simulink model "PhaseII_opalrt_NoProtection"  (Simulink 8.8)
settings: Solver=ode3  StartTime=0.0  StopTime=inf  FixedStep=Ts  RelTol=1e-5  EnableMultiTasking=on
PostLoadFcn:
  | %BESS ctrl
  | Kpf=0.005*3*12;
  | Kif=5*6;
  | 
  | Kpf1=0.005*3*12;
  | Kif1=5*6;
  | Kp_v=0.016*15*35;
  | Ki_v=12*25;
  | 
  | Kp_v1=0.016*15*35;
  | Ki_v1=12*25;
  | 
  | Vabc_B=12.47e3;
  | Vdc_ref=Vabc_B*2;
  | Kpwm=sqrt(2)*Vabc_B/Vdc_ref;
  | ZB=Vabc_B^2/1e6;
  | R=0.005*ZB;
  | Ibasefull=673/2*sqrt(2);
  | 
  | 
  | Ts_Control=1e-4;
  | ts=0.05;
  | delay=0.2;
  | offset=10e3;
  | t_plan=60;
  | t_monitor=.2;
  | t_mon=t_monitor;
  | scalingfactor=1;
  | x=0.5;
  | n=6;
  | %t_plan=1/15;
  | %t_monitor=10/900;
  | %t_mon=10/900;
  | 
  | %t_plan=1/5;
  | %t_monitor=10/300;
  | %t_mon=10/300;
  | %scalingfactor=1/300;
  | 
  | f0=60;
  | 
  | Pabc_B=1e6;
  | Iabc_B=Pabc_B*sqrt(2/3)/Vabc_B;  % pk value
  | Imax_1=2.5;
  | Ptrans_B=Pabc_B*200;
  | 
  | Vdc_ref=Vabc_B*2;
  | 
  | ZB=Vabc_B^2/Pabc_B;
  | L=0.1*ZB/2/pi/60;
  | R=0.1*ZB;
  | C=1/(4*pi^2*(2e3)^2*L);
  | 
  | LL=0.005*ZB/2/pi/60;
  | RR=0.005*ZB;
  | 
  | RC=0.02;
  | 
  | %%% Initial SOC %%%%
  | SOC_ini_BESS1=0.5;
  | ... (+223 lines)
InitFcn:
  | %BESS ctrl
  | Kpf=0.005*3*12;
  | Kif=5*6;
  | 
  | Kpf1=0.005*3*12;
  | Kif1=5*6;
  | Kp_v=0.016*15*35;
  | Ki_v=12*25;
  | 
  | Kp_v1=0.016*15*35;
  | Ki_v1=12*25;
  | 
  | Vabc_B=12.47e3;
  | Vdc_ref=Vabc_B*2;
  | Kpwm=sqrt(2)*Vabc_B/Vdc_ref;
  | ZB=Vabc_B^2/1e6;
  | R=0.005*ZB;
  | Ibasefull=673/2*sqrt(2);
  | 
  | 
  | Ts_Control=1e-4;
  | ts=0.05;
  | delay=0.2;
  | offset=10e3;
  | t_plan=60;
  | t_monitor=.2;
  | t_mon=t_monitor;
  | scalingfactor=1;
  | x=0.5;
  | n=6;
  | %t_plan=1/15;
  | %t_monitor=10/900;
  | %t_mon=10/900;
  | 
  | %t_plan=1/5;
  | %t_monitor=10/300;
  | %t_mon=10/300;
  | %scalingfactor=1/300;
  | 
  | f0=60;
  | 
  | Pabc_B=1e6;
  | Iabc_B=Pabc_B*sqrt(2/3)/Vabc_B;  % pk value
  | Imax_1=2.5;
  | Ptrans_B=Pabc_B*200;
  | 
  | Vdc_ref=Vabc_B*2;
  | 
  | ZB=Vabc_B^2/Pabc_B;
  | L=0.1*ZB/2/pi/60;
  | R=0.1*ZB;
  | C=1/(4*pi^2*(2e3)^2*L);
  | 
  | LL=0.005*ZB/2/pi/60;
  | RR=0.005*ZB;
  | 
  | RC=0.02;
  | 
  | %%% Initial SOC %%%%
  | SOC_ini_BESS1=0.5;
  | ... (+223 lines)
undefined symbols (not defined in the file): D1, Delta, DiscIntNeverNeededParam, Left, PG2ref, type, V
libraries: powerlib x220, powerlib_meascontrol x82, dspstat3 x54, dsparch4 x43, dspswit3 x24, simulink x19, simulink_extras x12, powerlib_extras x11, ssn_lib x7, artemis x6, rtlab x5, rtio_generic_dnp3 x5
(part 8 of 9)

== system PhaseII_opalrt_NoProtection/SS_LocalControl/BESS2/Sequence decomposition2 ==
  abc : Inport
  Phase : Inport  Port=2
  Add : Sum  Inputs=+++
  Add1 : Sum
  Add2 : Sum  Inputs=+-
  Add3 : Sum
  Add4 : Sum  Inputs=-+
  Alpha-Beta-Zero to dq0 : powerlib_meascontrol/Transformations/Alpha-Beta-Zero to dq0  Alignment=90 degrees behind phase A axis
  Alpha-Beta-Zero to dq1 : powerlib_meascontrol/Transformations/Alpha-Beta-Zero to dq0  Alignment=90 degrees behind phase A axis
  Delay : Delay  DelayLength=42  InitialCondition=0
  Delay1 : Delay  DelayLength=42  InitialCondition=0
  Demux1 : Demux  Outputs=2
  Demux4 : Demux  Outputs=3
  Fcn3 : Fcn  Expr=sqrt(2/3)*(u[1]-u[2]*1/2-u[3]*1/2)
  Fcn5 : Fcn  Expr=sqrt(2/3)*(u[2]*sqrt(3)/2-u[3]*sqrt(3)/2)
  Gain1 : Gain  Gain=-1
  Gain2 : Gain  Gain=1/3
  Gain3 : Gain
  Gain{6..9} (4 alike) : Gain  Gain=1/2
  Mux : Mux  Inputs=3
  Mux1 : Mux  Inputs=3
  Mux2 : Mux  Inputs=2
  Mux3 : Mux  Inputs=3
  Pos_dq : Outport
  Neg_dq : Outport  Port=2
  zero : Outport  Port=3
  wires:
  Demux1/1 -> Add2/1, Add3/1, Delay/1
  Mux2/1 -> Demux1/1
  Demux1/2 -> Delay1/1, Add4/2, Add1/1
  Mux/1 -> Alpha-Beta-Zero to dq1/1
  Gain1/1 -> Alpha-Beta-Zero to dq1/2
  Alpha-Beta-Zero to dq0/1 -> Pos_dq/1
  Alpha-Beta-Zero to dq1/1 -> Neg_dq/1
  abc/1 -> Demux4/1
  Demux4/1 -> Mux1/1, Add/1
  Demux4/2 -> Mux1/2, Add/3
  Demux4/3 -> Mux1/3, Add/2
  Delay1/1 -> Add2/2, Add3/2
  Delay/1 -> Add4/1, Add1/2
  Add1/1 -> Gain7/1
  Add2/1 -> Gain6/1
  Add4/1 -> Gain9/1
  Add3/1 -> Gain8/1
  Gain8/1 -> Mux/1
  Gain9/1 -> Mux/2
  Mux3/1 -> Alpha-Beta-Zero to dq0/1
  Gain6/1 -> Mux3/1
  Gain7/1 -> Mux3/2
  Add/1 -> Gain2/1, Gain3/1
  Gain2/1 -> zero/1
  Phase/1 -> Gain1/1, Alpha-Beta-Zero to dq0/2
  Gain3/1 -> Mux3/3, Mux/3
  Mux1/1 -> Fcn3/1, Fcn5/1
  Fcn3/1 -> Mux2/1
  Fcn5/1 -> Mux2/2

== system PhaseII_opalrt_NoProtection/SS_LocalControl/BESS2/Subsystem ==
  I_RMS : Inport
  Add : Sum  Inputs=+-
  Constant : Constant  Value=SOC_ini_BESS2*AH*3600
  Constant1 : Constant
  Gain : Gain  Gain=1/3600
  Gain3 : Gain  Gain=1/(AH*3600)
  Gain8 : Gain
  Integrator : Integrator
  Integrator1 : Integrator  InitialConditionSource=external  LimitOutput=on  UpperSaturationLimit=AH*3600  LowerSaturationLimit=0
  Battery_Ah : Outport
  Battery_SOC : Outport  Port=2
  wires:
  Gain8/1 -> Battery_SOC/1
  Gain/1 -> Battery_Ah/1
  I_RMS/1 -> Integrator1/1, Integrator/1
  Constant/1 -> Integrator1/2
  Add/1 -> Gain8/1
  Constant1/1 -> Add/1
  Gain3/1 -> Add/2
  Integrator1/1 -> Gain3/1
  Integrator/1 -> Gain/1

== system PhaseII_opalrt_NoProtection/SS_LocalControl/BESS2/V_theta_generation ==
  Pin : Inport
  Qin : Inport  Port=2
  Pin1 : Inport  Port=3
  "  " : Constant  Value=2*pi
  2 kHz1 : dsparch4/Analog Filter Design  method=Butterworth  filttype=Lowpass  N=2  Wlo=2*pi*0.1  Whi=80  Rp=2  Rs=40
  Constant1 : Constant  Value=1.64368  OutDataTypeStr=single
  D1 : Scope  Commented=on
  D{2..7} (6 alike) : Scope
  Delay : Delay  DelayLength=1  SampleTime=Ts
  Gain1 : Gain
  Gain2 : Gain  Gain=2*pi
  Gain3 : Gain
  Gain4 : Gain  Gain=1/2/pi
  Gain5 : Gain  Gain=1/2/pi
  Gain6 : Gain  Gain=0
  Gain7 : Gain  Gain=1/2/pi
  Gain8 : Gain  Gain=0
  Integrator : Integrator  ExternalReset=rising  InitialConditionSource=external  LimitOutput=on
  Kv : Constant  Value=0.1
  Math Function : Math  Operator=mod  SaturateOnIntegerOverflow=on
  P1 : Constant  Value=0.5
  P4 : Constant  Value=0
  P5 : Constant  Value=0.01
  Product : Product
  Product1 : Product
  Product2 : Product
  Q : Constant  Value=0
  Sum1 : Sum  Inputs=|-+
  Sum10 : Sum  Inputs=|++
  Sum13 : Sum  Inputs=+++
  Sum2 : Sum  Inputs=++++
  Sum3 : Sum  Inputs=|-+
  Sum4 : Sum
  V : Constant
  intergral : DiscreteTransferFcn  Commented=on  Numerator=Ts_Control/10  Denominator=[1 -1]  SampleTime=Ts_Control/10
  w0 : Constant  Value=60*2*pi
  w2 : Constant  Value=0
  Magd : Outport
  theta : Outport  Port=2
  Magq : Outport  Port=3
  frequency : Outport  Port=4
  tag scope: Phase_islanded_ref1=global
  wires:
  Sum10/1 -> Product/2
  w0/1 -> Sum13/1
  Gain4/1 -> frequency/1, D7/1
  Product/1 -> Gain2/1
  [Pba_ref2] -> Sum10/1
  Sum13/1 -> Integrator/1, Gain4/1
  "  "/1 -> Math Function/2
  Math Function/1 -> D3/1, theta/1
  Gain3/1 -> Gain8/1, Sum10/2
  Pin/1 -> Gain3/1
  Integrator/1 -> D5/1, [Phase_islanded_ref1], Math Function/1
  P1/1 -> Product/1
  Gain2/1 -> Sum13/2
  Gain1/1 -> Sum2/2
  Kv/1 -> Product1/1
  Sum1/1 -> Product1/2
  Sum2/1 -> D2/1, Magd/1, Gain5/1
  V/1 -> Sum2/1
  Q/1 -> Sum1/1
  Product1/1 -> Gain1/1
  Qin/1 -> Sum3/2, Sum1/2
  Gain6/1 -> Sum4/2
  Product2/1 -> Gain6/1
  P5/1 -> Product2/1
  Sum3/1 -> Product2/2
  Sum4/1 -> D4/1, Magq/1, Gain7/1
  P4/1 -> Sum3/1
  w2/1 -> Sum4/1
  Pin1/1 -> Integrator/2
  [Phase_grid2] -> Delay/1
  Delay/1 -> Integrator/3
  [Fba_ref2] -> Sum13/3
  [Vba_ref2] -> Sum2/3
  Gain8/1 -> 2 kHz1/1
  2 kHz1/1 -> Sum2/4

== system PhaseII_opalrt_NoProtection/SS_LocalControl/PV2/LPF1 ==
  In1 : Inport
  2 kHz : dsparch4/Analog Filter Design  method=Butterworth  filttype=Lowpass  N=2  Wlo=2*pi*100  Whi=80  Rp=2  Rs=40
  2 kHz1 : dsparch4/Analog Filter Design  method=Butterworth  filttype=Lowpass  N=2  Wlo=2*pi*100  Whi=80  Rp=2  Rs=40
  Demux : Demux  Outputs=2
  Mux : Mux  Inputs=2
  Out1 : Outport
  wires:
  Mux/1 -> Out1/1
  In1/1 -> Demux/1
  Demux/1 -> 2 kHz/1
  2 kHz/1 -> Mux/1
  2 kHz1/1 -> Mux/2
  Demux/2 -> 2 kHz1/1

== system PhaseII_opalrt_NoProtection/SS_LocalControl/PV2/PI_daxis1 ==
  Error : Inport
  Add : Sum
  Constant1 : Constant  Value=10  OutDataTypeStr=single
  Constant2 : Constant  Value=-10  OutDataTypeStr=single
  Constant3 : Constant  Value=0  OutDataTypeStr=single
  Embedded MATLAB Function1 : MATLAB Function  TreatAsAtomicUnit=on
  Integrator : Integrator
  K : Gain  Gain=Iabc_B
  Ki1 : Gain  Gain=Ki_I_PV
  Kp1 : Gain  Gain=Kp_I_PV
  Logical Operator : Logic  AllPortsSameDT=off  OutDataTypeStr=boolean
  Relational Operator : RelationalOperator  Operator=<  OutDataTypeStr=boolean  RndMeth=Nearest
  Relational Operator1 : RelationalOperator  Operator=>  OutDataTypeStr=boolean  RndMeth=Nearest
  Saturation : Saturate  UpperLimit=10  LowerLimit=-10
  Switch : Switch  Threshold=.5
  Out : Outport
  wires:
  Kp1/1 -> Add/1
  Relational Operator/1 -> Logical Operator/1
  Relational Operator1/1 -> Logical Operator/2
  Saturation/1 -> Out/1
  Constant1/1 -> Relational Operator/2
  Constant2/1 -> Relational Operator1/2
  Logical Operator/1 -> Embedded MATLAB Function1/2(enable)
  Embedded MATLAB Function1/1(dout) -> Integrator/1
  Add/1 -> Relational Operator/1, Relational Operator1/1, Saturation/1
  Error/1 -> K/1
  K/1 -> Kp1/1, Ki1/1
  [PV1_En] -> Switch/2
  Constant3/1 -> Switch/3
  Switch/1 -> Embedded MATLAB Function1/1(din)
  Ki1/1 -> Switch/1
  Integrator/1 -> Add/2

== system PhaseII_opalrt_NoProtection/SS_LocalControl/PV2/PI_daxis2 ==
  Error : Inport
  Add : Sum
  Constant1 : Constant  Value=10  OutDataTypeStr=single
  Constant2 : Constant  Value=-10  OutDataTypeStr=single
  Constant3 : Constant  Value=0  OutDataTypeStr=single
  Embedded MATLAB Function1 : MATLAB Function  TreatAsAtomicUnit=on
  Integrator : Integrator  InitialCondition=0.069585
  K : Gain  Gain=Iabc_B
  Ki1 : Gain  Gain=Ki_I_PV
  Kp1 : Gain  Gain=Kp_I_PV
  Logical Operator : Logic  AllPortsSameDT=off  OutDataTypeStr=boolean
  Relational Operator : RelationalOperator  Operator=<  OutDataTypeStr=boolean  RndMeth=Nearest
  Relational Operator1 : RelationalOperator  Operator=>  OutDataTypeStr=boolean  RndMeth=Nearest
  Saturation : Saturate  UpperLimit=10  LowerLimit=-10
  Switch : Switch  Threshold=.5
  Out : Outport
  wires:
  Ki1/1 -> Switch/1
  Switch/1 -> Embedded MATLAB Function1/1(din)
  Constant3/1 -> Switch/3
  [PV1_En] -> Switch/2
  K/1 -> Ki1/1, Kp1/1
  Error/1 -> K/1
  Add/1 -> Saturation/1, Relational Operator1/1, Relational Operator/1
  Embedded MATLAB Function1/1(dout) -> Integrator/1
  Logical Operator/1 -> Embedded MATLAB Function1/2(enable)
  Constant2/1 -> Relational Operator1/2
  Constant1/1 -> Relational Operator/2
  Saturation/1 -> Out/1
  Relational Operator1/1 -> Logical Operator/2
  Relational Operator/1 -> Logical Operator/1
  Kp1/1 -> Add/1
  Integrator/1 -> Add/2

== system PhaseII_opalrt_NoProtection/SS_LocalControl/PV2/PLL  ==
  Vabc_CL1 : Inport
  3-phase PLL1 : Subsystem  AncestorBlock="powerlib_extras/Control  Blocks/3-phase PLL"  DialogController=POWERSYS.PowerSysDialog  mask(3-phase PLL){Par_Init=[0 60], ParK=[ 53 900 0]*5, AGC=off}
      mask prompts: Par_Init "Initial inputs:[ Phase(degrees)   Frequency(Hz) ]"; ParK "Regulator gains [ Kp  Ki  Kd ]"; AGC "Enable Automatic Gain Control"
      mask help:
      | This Phase Locked Loop (PLL) system can be used  to synchronize on a set of variable frequency, three-phase sinusoidal signals. If the Automatic Gain Control is enabled, the input (phase error) of the PLL regulator is scaled according to the input signal magnitude.
      |
      | For optimal performance, the following settings are recommended:
      |   [ Kp Ki  Kd ] = [ 180  3200  1 ]
      |   "Enable Automatic Gain Control" checked
      |
      | Input 1: Vector containing the normalized three-phase signals [Va Vb Vc]
      | Output 1:  Measured frequency (Hz) = w/(2pi)
      | Output 2:  Ramp w.t varying between  0 and 2*pi,
      |      synchronized on zero crossings of the fundamental (positive-sequence) of phase A.
      | Output 3: Vector [sin(wt) cos(wt)]
      mask init:
      | a=exp(j*2*pi/3);
      | a2=exp(-j*2*pi/3);
      | Kp=ParK(1);
      | Ki=ParK(2);
      | if length(ParK)==2
      |     Kd=0;
      | else
      |     Kd=ParK(3);
      | end  
      | Phase_Init=Par_Init(1);
      | Finit=Par_Init(2);
      | power_initmask();
      mask Help: This block is part of a subset of blocks in the Extras library that does not have documentation associated with it, other than the block mask description.
      mask Display: disp('')
  Demux : Demux  Outputs=3
  SW_Local1 : Scope  NumInputPorts=3
  VLtoVphase6 : Subsystem
  sin_cos : Outport
  vd : Outport  Port=2
  vq : Outport  Port=3
  tag scope: f_PV1=global
  wires:
  3-phase PLL1/3(Sin_Cos) -> sin_cos/1
  Vabc_CL1/1 -> VLtoVphase6/1(VLabc)
  VLtoVphase6/1(Vph_abc) -> [Vph_PV1]
  Demux/2 -> vq/1
  Demux/1 -> vd/1
  3-phase PLL1/4(Vdq0) -> SW_Local1/3, Demux/1
  3-phase PLL1/1(Freq) -> SW_Local1/1, [f_PV1]
  [Vph_PV1] -> 3-phase PLL1/1(Vabc (pu)), SW_Local1/2

== system PhaseII_opalrt_NoProtection/SS_LocalControl/PV2/SW Command ==
  f : Inport
  Vd : Inport  Port=2
  SW_Ctr : Inport  Port=3
  "   3" : UnitDelay  SampleTime=Ts
  Abs2 : Abs
  Abs3 : Abs
  Add3 : Sum  Inputs=+-
  Add4 : Sum  Inputs=+-
  Constant1 : Constant  Value=2
  Constant20 : Constant  Value=.1
  Constant21 : Constant  Value=.5
  Constant22 : Constant
  Constant23 : Constant  Value=f0
  Conv : DataTypeConversion  OutDataTypeStr=double
  Counter : dspswit3/Counter  Direction=Up  CountEvent=Non-zero sample  CounterSize=User defined  MaxCount=255  InitialCount=0  Output=Hit  HitValue=50  ResetInput=on  SamplesPerFrame=1  Ts=1  CntDtype=double  HitDtype=Logical
  Counter1 : dspswit3/Counter  Direction=Up  CountEvent=Rising edge  CounterSize=User defined  MaxCount=255  InitialCount=0  Output=Count  HitValue=50  ResetInput=off  SamplesPerFrame=1  Ts=1  CntDtype=double  HitDtype=Logical
  D Latch2 : simulink_extras/Flip Flops/D Latch
  Logical Operator : Logic  AllPortsSameDT=off  OutDataTypeStr=boolean
  Logical Operator1 : Logic  Operator=NOT  AllPortsSameDT=off  OutDataTypeStr=boolean
  Logical Operator4 : Logic  AllPortsSameDT=off  OutDataTypeStr=boolean
  Relational Operator1 : RelationalOperator  OutDataTypeStr=boolean  RndMeth=Nearest
  Relational Operator2 : RelationalOperator  Operator=<=  OutDataTypeStr=boolean  RndMeth=Nearest
  Relational Operator3 : RelationalOperator  Operator=<=  OutDataTypeStr=boolean  RndMeth=Nearest
  SW_Cmd : Outport
  wires:
  Abs2/1 -> Relational Operator2/1
  Vd/1 -> Add4/1
  Add3/1 -> Abs2/1
  Constant23/1 -> Add3/2
  Constant21/1 -> Relational Operator2/2
  Relational Operator2/1 -> Logical Operator4/1
  Add4/1 -> Abs3/1
  Constant22/1 -> Add4/2
  D Latch2/1 -> Logical Operator/1
  Relational Operator3/1 -> Logical Operator4/2
  Abs3/1 -> Relational Operator3/1
  Constant20/1 -> Relational Operator3/2
  f/1 -> Add3/1
  SW_Ctr/1 -> Logical Operator/2
  Logical Operator/1 -> Conv/1
  Relational Operator1/1 -> D Latch2/1
  D Latch2/2 -> "   3"/1
  "   3"/1 -> D Latch2/2
  Constant1/1 -> Relational Operator1/2
  Counter/1 -> Counter1/1
  Counter1/1 -> Relational Operator1/1
  Logical Operator1/1 -> Counter/2
  Logical Operator4/1 -> Logical Operator1/1, Counter/1
  Conv/1 -> SW_Cmd/1

== system PhaseII_opalrt_NoProtection/SS_LocalControl/PV2/Subsystem2 ==
  Dabc : Inport
  Add : Sum  Inputs=+-
  Add1 : Sum  Inputs=-+
  Add{2..5} (4 alike) : Sum
  Constant : Constant
  Constant1 : Constant  Value=-1
  Demux1 : Demux  Outputs=3
  Demux5 : Demux  Outputs=3
  Demux6 : Demux  Outputs=3
  Gain2 : Gain  Gain=0.5
  MinMax : MinMax  Function=max  Inputs=3
  MinMax1 : MinMax  Inputs=3
  Mux : Mux  Inputs=3
  abc : Outport
  wires:
  Mux/1 -> abc/1
  Dabc/1 -> Demux1/1, Demux5/1, [Dabc]
  Add5/1 -> Mux/3
  Add4/1 -> Mux/2
  Add3/1 -> Mux/1
  [m_cm] -> Add5/2
  Demux6/3 -> Add5/1
  Demux6/2 -> Add4/2
  [m_cm] -> Add4/1
  [m_cm] -> Add3/1
  Demux6/1 -> Add3/2
  [Dabc] -> Demux6/1
  Gain2/1 -> [m_cm]
  Add2/1 -> Gain2/1
  Add1/1 -> Add2/2
  Add/1 -> Add2/1
  Constant1/1 -> Add1/2
  MinMax1/1 -> Add1/1
  Constant/1 -> Add/1
  MinMax/1 -> Add/2
  Demux5/3 -> MinMax1/3
  Demux5/1 -> MinMax1/1
  Demux5/2 -> MinMax1/2
  Demux1/3 -> MinMax/3
  Demux1/1 -> MinMax/1
  Demux1/2 -> MinMax/2

== system PhaseII_opalrt_NoProtection/SM_System/Generator2/Intelliupter Measurement4/3Pto1P1 ==
  Vabc : Inport
  Demux9 : Demux  Outputs=3
  Gain : Gain  Gain=sqrt(2)
  Gain1 : Gain  Gain=sqrt(2)
  Gain2 : Gain  Gain=sqrt(2)
  Moving RMS : dspstat3/Moving RMS  Method=Exponential weighting  SpecifyWindowLength=off  WindowLength=4  ForgettingFactor=0.999  SimulateUsing=Code generation
  Moving RMS1 : dspstat3/Moving RMS  Method=Exponential weighting  SpecifyWindowLength=off  WindowLength=4  ForgettingFactor=0.999  SimulateUsing=Code generation
  Moving RMS2 : dspstat3/Moving RMS  Method=Exponential weighting  SpecifyWindowLength=off  WindowLength=4  ForgettingFactor=0.999  SimulateUsing=Code generation
  Va : Outport
  Vb : Outport  Port=2
  Vc : Outport  Port=3
  wires:
  Gain2/1 -> Vc/1
  Moving RMS2/1 -> Gain2/1
  Gain1/1 -> Vb/1
  Moving RMS1/1 -> Gain1/1
  Gain/1 -> Va/1
  Moving RMS/1 -> Gain/1
  Vabc/1 -> Demux9/1
  Demux9/2 -> Moving RMS1/1
  Demux9/1 -> Moving RMS/1
  Demux9/3 -> Moving RMS2/1

== system PhaseII_opalrt_NoProtection/SM_System/Generator2/Intelliupter Measurement4/3Pto1P2 ==
  Vabc : Inport
  Demux9 : Demux  Outputs=3
  Gain : Gain  Gain=sqrt(2)
  Gain1 : Gain  Gain=sqrt(2)
  Gain2 : Gain  Gain=sqrt(2)
  Moving RMS : dspstat3/Moving RMS  Method=Exponential weighting  SpecifyWindowLength=off  WindowLength=4  ForgettingFactor=0.999  SimulateUsing=Code generation
  Moving RMS1 : dspstat3/Moving RMS  Method=Exponential weighting  SpecifyWindowLength=off  WindowLength=4  ForgettingFactor=0.999  SimulateUsing=Code generation
  Moving RMS2 : dspstat3/Moving RMS  Method=Exponential weighting  SpecifyWindowLength=off  WindowLength=4  ForgettingFactor=0.999  SimulateUsing=Code generation
  Va : Outport
  Vb : Outport  Port=2
  Vc : Outport  Port=3
  wires:
  Demux9/3 -> Moving RMS2/1
  Demux9/1 -> Moving RMS/1
  Demux9/2 -> Moving RMS1/1
  Vabc/1 -> Demux9/1
  Moving RMS/1 -> Gain/1
  Gain/1 -> Va/1
  Moving RMS1/1 -> Gain1/1
  Gain1/1 -> Vb/1
  Moving RMS2/1 -> Gain2/1
  Gain2/1 -> Vc/1

== system PhaseII_opalrt_NoProtection/SM_System/Generator2/Intelliupter Measurement4/Detection ==
  V : Inport
  I : Inport  Port=2
  Abs2 : Abs
  Constant4 : Constant  Value=10  SampleTime=-1
  Constant5 : Constant  Value=0  SampleTime=-1
  Constant6 : Constant  SampleTime=-1
  Constant8 : Constant  Value=-1  SampleTime=-1
  Demux : Demux  Commented=on  Outputs=3
  Power : powerlib_meascontrol/Measurements/Power  Freq=60  Vinit=[1, 0]  Iinit=[1, 0]  Ts=0
  Relational Operator3 : RelationalOperator  Operator=<  OutDataTypeStr=boolean  RndMeth=Simplest
  Scope : Scope
  Sum : Sum  Commented=on  Inputs=+++
  Sum of Elements : Sum  Inputs=+
  Switch : Switch  Criteria=u2 > Threshold  Threshold=0.5
  Switch2 : Switch  Criteria=u2 > Threshold
  Terminator : Terminator
  Direction : Outport
  wires:
  Power/2 -> Terminator/1
  I/1 -> Power/2
  V/1 -> Power/1
  Switch2/1 -> Switch/3
  Constant5/1 -> Switch2/3
  Relational Operator3/1 -> Switch/2
  Constant6/1 -> Switch2/1
  Constant8/1 -> Switch/1
  Demux/3 -> Sum/3
  Demux/1 -> Sum/1
  Demux/2 -> Sum/2
  Switch/1 -> Direction/1
  Abs2/1 -> Relational Operator3/1
  Constant4/1 -> Relational Operator3/2
  Power/1 -> Sum of Elements/1
  Sum of Elements/1 -> Switch2/2, Scope/1, Abs2/1

== system PhaseII_opalrt_NoProtection/SM_System/Generator2/Intelliupter Measurement4/Subsystem ==
  VaL : Inport
  VaR : Inport  Port=2
  VbL : Inport  Port=3
  VbR : Inport  Port=4
  VcL : Inport  Port=5
  VcR : Inport  Port=6
  Constant7 : Constant  Value=8e3
  Logical Operator : Logic  Inputs=3  AllPortsSameDT=off  OutDataTypeStr=boolean
  Relational Operator : RelationalOperator  Operator=<=  OutDataTypeStr=boolean  RndMeth=Simplest
  Relational Operator6 : RelationalOperator  Operator=<=  OutDataTypeStr=boolean  RndMeth=Simplest
  Relational Operator7 : RelationalOperator  Operator=<=  OutDataTypeStr=boolean  RndMeth=Simplest
  Subtract1 : Sum  Inputs=+-
  Subtract3 : Sum  Inputs=+-
  Subtract4 : Sum  Inputs=+-
  Vdiff : Outport
  wires:
  Subtract4/1 -> Relational Operator7/1
  Subtract3/1 -> Relational Operator6/1
  Constant7/1 -> Relational Operator7/2, Relational Operator6/2, Relational Operator/2
  Subtract1/1 -> Relational Operator/1
  VcR/1 -> Subtract4/2
  Relational Operator7/1 -> Logical Operator/3
  VcL/1 -> Subtract4/1
  VbL/1 -> Subtract3/1
  VbR/1 -> Subtract3/2
  Relational Operator/1 -> Logical Operator/1
  VaL/1 -> Subtract1/1
  VaR/1 -> Subtract1/2
  Relational Operator6/1 -> Logical Operator/2
  Logical Operator/1 -> Vdiff/1

== system PhaseII_opalrt_NoProtection/SM_System/Generator2/Intelliupter Measurement4/Subsystem1 ==
  VaL : Inport
  VbL : Inport  Port=2
  VcL : Inport  Port=3
  VaR : Inport  Port=4
  VbR : Inport  Port=5
  VcR : Inport  Port=6
  Constant7 : Constant  Value=1e3
  Logical Operator : Logic  Inputs=3  AllPortsSameDT=off  OutDataTypeStr=boolean
  Logical Operator1 : Logic  Inputs=3  AllPortsSameDT=off  OutDataTypeStr=boolean
  Relational Operator{3..4,6..9} (6 alike) : RelationalOperator  Operator=<=  OutDataTypeStr=boolean  RndMeth=Simplest
  VL : Outport
  VR : Outport  Port=2
  wires:
  Constant7/1 -> Relational Operator9/2, Relational Operator8/2, Relational Operator4/2, Relational Operator3/2, Relational Operator7/2, Relational Operator6/2
  VcL/1 -> Relational Operator4/1
  VaR/1 -> Relational Operator3/1
  Relational Operator4/1 -> Logical Operator/3
  Relational Operator6/1 -> Logical Operator/2
  VaL/1 -> Relational Operator7/1
  Relational Operator3/1 -> Logical Operator1/1
  VbL/1 -> Relational Operator6/1
  VcR/1 -> Relational Operator8/1
  Relational Operator9/1 -> Logical Operator1/2
  VbR/1 -> Relational Operator9/1
  Relational Operator7/1 -> Logical Operator/1
  Relational Operator8/1 -> Logical Operator1/3
  Logical Operator/1 -> VL/1
  Logical Operator1/1 -> VR/1

== system PhaseII_opalrt_NoProtection/SM_System/Generator2/Subsystem2/Exciter ==
  Vt : Inport
  Vtr0 : Inport  Port=2
  Vpss : Inport  Port=3
  Add : Sum  Inputs=++-
  Saturation : Saturate  UpperLimit=Efdmax  LowerLimit=0  ZeroCross=off
  Transfer Fcn : TransferFcn  Numerator=[KA/10]  Denominator=[TA*10 1]
  Ef : Outport
  wires:
  Vpss/1 -> Add/2
  Vt/1 -> Add/3
  Add/1 -> Transfer Fcn/1
  Transfer Fcn/1 -> Saturation/1
  Vtr0/1 -> Add/1
  Saturation/1 -> Ef/1

== system PhaseII_opalrt_NoProtection/SM_System/Generator2/Subsystem2/PSS ==
  dw : Inport
  Gain : Gain  Gain=100
  Transfer Fcn : TransferFcn  Numerator=[10 0]  Denominator=[10 1]
  Transfer Fcn1 : TransferFcn  Numerator=[0.9606 1]  Denominator=[0.1648 1]
  Transfer Fcn2 : TransferFcn  Numerator=[3 1]  Denominator=[5.4 1]
  Transfer Fcn3 : TransferFcn  Numerator=[0.1648 1]  Denominator=[0.9606 1]
  Transfer Fcn4 : TransferFcn  Numerator=[0.3053 1]  Denominator=[0.5185 1]
  Transfer Fcn5 : TransferFcn  Numerator=[0.3053 1]  Denominator=[0.5185 1]
  Vpss : Outport
  wires:
  dw/1 -> Gain/1
  Gain/1 -> Transfer Fcn/1
  ? -> ?
  Transfer Fcn/1 -> Transfer Fcn4/1
  Transfer Fcn4/1 -> Transfer Fcn5/1
  Transfer Fcn5/1 -> Vpss/1

== system PhaseII_opalrt_NoProtection/SM_System/Generator2/Subsystem2/thermal_turbine_droop ==
  dw : Inport
  pe : Inport  Port=2
  Constant1 : Constant  Commented=on  Value=PG2ref
  Dead Zone : DeadZone  LowerValue=-0.05  UpperValue=0.05  SaturateOnIntegerOverflow=on
  Governor : TransferFcn  Denominator=[TG 1]
  Saturation : Saturate  UpperLimit=2  LowerLimit=0  ZeroCross=off
  Saturation1 : Saturate  UpperLimit=0.2  LowerLimit=-0.2  ZeroCross=off
  Sum : Sum  Inputs=+-+
  Sum1 : Sum  Inputs=++-
  droop : Gain  Gain=R_1
  droop1 : Gain  Gain=0
  inertial : TransferFcn  Denominator=[M2 D]
  turbine : TransferFcn  Numerator=[FHP*TRH 1]  Denominator=[TRH*TCH TRH+TCH 1]
  dww : Outport
  wires:
  dw/1 -> droop/1
  turbine/1 -> Saturation/1
  Sum1/1 -> inertial/1
  Governor/1 -> turbine/1
  Sum/1 -> Governor/1
  Saturation/1 -> Sum1/2
  [Gen_P_out] -> Sum1/1
  [Gen_F] -> Sum/1
  inertial/1 -> droop1/1, Saturation1/1
  [Gen_P] -> Sum/3
  Saturation1/1 -> dww/1
  droop1/1 -> Sum/2
  pe/1 -> Sum1/3

== system PhaseII_opalrt_NoProtection/SM_System/Generator2/Subsystem2/thermal_turbine_droop1 ==
  dw : Inport
  pe : Inport  Port=2
  Constant1 : Constant  Commented=on  Value=PG2ref
  Governor : TransferFcn  Denominator=[TG 1]
  Sum : Sum  Inputs=|-+
  Sum1 : Sum  Inputs=++-
  droop : Gain  Gain=R_1
  inertial : TransferFcn  Denominator=[M1 D]
  turbine : TransferFcn  Numerator=[FHP*TRH 1]  Denominator=[TRH*TCH TRH+TCH 1]
  dww : Outport
  wires:
  [Gen_P_out] -> Sum/2
  Governor/1 -> turbine/1
  inertial/1 -> dww/1
  Sum1/1 -> inertial/1
  pe/1 -> Sum1/3
  turbine/1 -> Sum1/2
  dw/1 -> droop/1
  droop/1 -> Sum/1
  Sum/1 -> Governor/1

== system PhaseII_opalrt_NoProtection/SM_System/Generator2/abc -> dq/abc -> dq ==
  a : Inport
  b : Inport  Port=2
  c : Inport  Port=3
  Theta : Inport  Port=4
  Add1 : Sum  Inputs=+++
  Add10 : Sum  Inputs=+++
  Add11 : Sum  Inputs=+++
  Add4 : Sum  Inputs=+-
  Add8 : Sum
  Constant6 : Constant  Value=2/3*pi
  Constant7 : Constant  Value=2/3*pi
  Divide{6..11} (6 alike) : Product  Inputs=**
  Gain1 : Gain  Gain=2/3
  Gain5 : Gain  Gain=2/3
  Gain6 : Gain  Gain=1/3
  Trigonometric Function : Trigonometry  Operator=cos
  Trigonometric Function1 : Trigonometry  Operator=cos
  Trigonometric Function2 : Trigonometry  Operator=cos
  Trigonometric Function3 : Trigonometry
  Trigonometric Function4 : Trigonometry
  Trigonometric Function5 : Trigonometry
  id : Outport
  iq : Outport  Port=2
  i0 : Outport  Port=3
  wires:
  Theta/1 -> Add4/1, Add8/1, Trigonometric Function/1, Trigonometric Function3/1  "wt"
  Constant6/1 -> Add4/2
  Add4/1 -> Trigonometric Function1/1, Trigonometric Function4/1
  Add8/1 -> Trigonometric Function2/1, Trigonometric Function5/1
  Trigonometric Function3/1 -> Divide7/2
  Trigonometric Function4/1 -> Divide9/2
  Trigonometric Function5/1 -> Divide11/2
  a/1 -> Divide6/1, Divide7/1, Add1/1
  Trigonometric Function/1 -> Divide6/2
  Trigonometric Function2/1 -> Divide10/2
  Trigonometric Function1/1 -> Divide8/2
  b/1 -> Divide8/1, Divide9/1, Add1/2
  c/1 -> Divide10/1, Divide11/1, Add1/3
  Constant7/1 -> Add8/2
  Divide6/1 -> Add10/1
  Divide8/1 -> Add10/2
  Divide10/1 -> Add10/3
  Divide7/1 -> Add11/1
  Divide9/1 -> Add11/2
  Divide11/1 -> Add11/3
  Add10/1 -> Gain1/1
  Add11/1 -> Gain5/1
  Gain1/1 -> id/1
  Gain5/1 -> iq/1
  Add1/1 -> Gain6/1
  Gain6/1 -> i0/1

== system PhaseII_opalrt_NoProtection/SM_System/Generator2/abc -> dq1/abc -> dq ==
  a : Inport
  b : Inport  Port=2
  c : Inport  Port=3
  Theta : Inport  Port=4
  Add1 : Sum  Inputs=+++
  Add10 : Sum  Inputs=+++
  Add11 : Sum  Inputs=+++
  Add4 : Sum  Inputs=+-
  Add8 : Sum
  Constant6 : Constant  Value=2/3*pi
  Constant7 : Constant  Value=2/3*pi
  Divide{6..11} (6 alike) : Product  Inputs=**
  Gain1 : Gain  Gain=2/3
  Gain5 : Gain  Gain=2/3
  Gain6 : Gain  Gain=2/3
  Trigonometric Function : Trigonometry  Operator=cos
  Trigonometric Function1 : Trigonometry  Operator=cos
  Trigonometric Function2 : Trigonometry  Operator=cos
  Trigonometric Function3 : Trigonometry
  Trigonometric Function4 : Trigonometry
  Trigonometric Function5 : Trigonometry
  id : Outport
  iq : Outport  Port=2
  i0 : Outport  Port=3
  wires:
  Theta/1 -> Add4/1, Add8/1, Trigonometric Function/1, Trigonometric Function3/1  "wt"
  Constant6/1 -> Add4/2
  Add4/1 -> Trigonometric Function1/1, Trigonometric Function4/1
  Add8/1 -> Trigonometric Function2/1, Trigonometric Function5/1
  Trigonometric Function3/1 -> Divide7/2
  Trigonometric Function4/1 -> Divide9/2
  Trigonometric Function5/1 -> Divide11/2
  a/1 -> Divide6/1, Divide7/1, Add1/1
  Trigonometric Function/1 -> Divide6/2
  Trigonometric Function2/1 -> Divide10/2
  Trigonometric Function1/1 -> Divide8/2
  b/1 -> Divide8/1, Divide9/1, Add1/2
  c/1 -> Divide10/1, Divide11/1, Add1/3
  Constant7/1 -> Add8/2
  Divide6/1 -> Add10/1
  Divide8/1 -> Add10/2
  Divide10/1 -> Add10/3
  Divide7/1 -> Add11/1
  Divide9/1 -> Add11/2
  Divide11/1 -> Add11/3
  Add10/1 -> Gain1/1
  Add11/1 -> Gain5/1
  Gain1/1 -> id/1
  Gain5/1 -> iq/1
  Add1/1 -> Gain6/1
  Gain6/1 -> i0/1

== system PhaseII_opalrt_NoProtection/SM_System/Generator2/dq -> abc/dq -> abc ==
  d : Inport
  q : Inport  Port=2
  Theta : Inport  Port=3
  Add1 : Sum  Inputs=+++
  Add10 : Sum  Inputs=+++
  Add11 : Sum  Inputs=+++
  Add4 : Sum  Inputs=+-
  Add8 : Sum
  Constant6 : Constant  Value=2/3*pi
  Constant7 : Constant  Value=2/3*pi
  Divide{6..11} (6 alike) : Product  Inputs=**
  Trigonometric Function : Trigonometry  Operator=cos
  Trigonometric Function1 : Trigonometry  Operator=cos
  Trigonometric Function2 : Trigonometry  Operator=cos
  Trigonometric Function3 : Trigonometry
  Trigonometric Function4 : Trigonometry
  Trigonometric Function5 : Trigonometry
  a : Outport
  b : Outport  Port=2
  c : Outport  Port=3
  wires:
  Add11/1 -> b/1
  Add10/1 -> a/1
  Divide9/1 -> Add11/2
  Divide6/1 -> Add10/1
  Constant7/1 -> Add8/2
  Trigonometric Function1/1 -> Divide8/2
  Trigonometric Function2/1 -> Divide10/2
  Trigonometric Function/1 -> Divide6/2
  Trigonometric Function5/1 -> Divide11/2
  Trigonometric Function4/1 -> Divide9/2
  Trigonometric Function3/1 -> Divide7/2
  Add8/1 -> Trigonometric Function5/1, Trigonometric Function2/1
  Add4/1 -> Trigonometric Function4/1, Trigonometric Function1/1
  Constant6/1 -> Add4/2
  Theta/1 -> Trigonometric Function3/1, Trigonometric Function/1, Add8/1, Add4/1  "wt"
  d/1 -> Divide6/1, Divide8/1, Divide10/1
  Add1/1 -> c/1
  Divide7/1 -> Add10/2
  q/1 -> Divide7/1, Divide9/1, Divide11/1
  Divide8/1 -> Add11/1
  Divide11/1 -> Add1/2
  Divide10/1 -> Add1/1

== system PhaseII_opalrt_NoProtection/SM_System/Intellirupter/Intelliupter Measurement1/3Pto1P1 ==
  Vabc : Inport
  Demux9 : Demux  Outputs=3
  Gain : Gain  Gain=sqrt(2)
  Gain1 : Gain  Gain=sqrt(2)
  Gain2 : Gain  Gain=sqrt(2)
  Moving RMS : dspstat3/Moving RMS  Method=Exponential weighting  SpecifyWindowLength=off  WindowLength=4  ForgettingFactor=0.999  SimulateUsing=Code generation
  Moving RMS1 : dspstat3/Moving RMS  Method=Exponential weighting  SpecifyWindowLength=off  WindowLength=4  ForgettingFactor=0.999  SimulateUsing=Code generation
  Moving RMS2 : dspstat3/Moving RMS  Method=Exponential weighting  SpecifyWindowLength=off  WindowLength=4  ForgettingFactor=0.999  SimulateUsing=Code generation
  Va : Outport
  Vb : Outport  Port=2
  Vc : Outport  Port=3
  wires:
  Demux9/3 -> Moving RMS2/1
  Demux9/1 -> Moving RMS/1
  Demux9/2 -> Moving RMS1/1
  Vabc/1 -> Demux9/1
  Moving RMS/1 -> Gain/1
  Gain/1 -> Va/1
  Moving RMS1/1 -> Gain1/1
  Gain1/1 -> Vb/1
  Moving RMS2/1 -> Gain2/1
  Gain2/1 -> Vc/1

== system PhaseII_opalrt_NoProtection/SM_System/Intellirupter/Intelliupter Measurement1/3Pto1P2 ==
  Vabc : Inport
  Demux9 : Demux  Outputs=3
  Gain : Gain  Gain=sqrt(2)
  Gain1 : Gain  Gain=sqrt(2)
  Gain2 : Gain  Gain=sqrt(2)
  Moving RMS : dspstat3/Moving RMS  Method=Exponential weighting  SpecifyWindowLength=off  WindowLength=4  ForgettingFactor=0.999  SimulateUsing=Code generation
  Moving RMS1 : dspstat3/Moving RMS  Method=Exponential weighting  SpecifyWindowLength=off  WindowLength=4  ForgettingFactor=0.999  SimulateUsing=Code generation
  Moving RMS2 : dspstat3/Moving RMS  Method=Exponential weighting  SpecifyWindowLength=off  WindowLength=4  ForgettingFactor=0.999  SimulateUsing=Code generation
  Va : Outport
  Vb : Outport  Port=2
  Vc : Outport  Port=3
  wires:
  Gain2/1 -> Vc/1
  Moving RMS2/1 -> Gain2/1
  Gain1/1 -> Vb/1
  Moving RMS1/1 -> Gain1/1
  Gain/1 -> Va/1
  Moving RMS/1 -> Gain/1
  Vabc/1 -> Demux9/1
  Demux9/2 -> Moving RMS1/1
  Demux9/1 -> Moving RMS/1
  Demux9/3 -> Moving RMS2/1

== system PhaseII_opalrt_NoProtection/SM_System/Intellirupter/Intelliupter Measurement1/Subsystem ==
  VaL : Inport
  VaR : Inport  Port=2
  VbL : Inport  Port=3
  VbR : Inport  Port=4
  VcL : Inport  Port=5
  VcR : Inport  Port=6
  Logical Operator : Logic  Inputs=3  AllPortsSameDT=off  OutDataTypeStr=boolean
  Relational Operator : RelationalOperator  Operator=<=  OutDataTypeStr=boolean  RndMeth=Simplest
  Relational Operator6 : RelationalOperator  Operator=<=  OutDataTypeStr=boolean  RndMeth=Simplest
  Relational Operator7 : RelationalOperator  Operator=<=  OutDataTypeStr=boolean  RndMeth=Simplest
  Subtract1 : Sum  Inputs=+-
  Subtract3 : Sum  Inputs=+-
  Subtract4 : Sum  Inputs=+-
  Vdiff : Outport
  wires:
  Logical Operator/1 -> Vdiff/1
  Relational Operator6/1 -> Logical Operator/2
  VaR/1 -> Subtract1/2
  VaL/1 -> Subtract1/1
  Relational Operator/1 -> Logical Operator/1
  VbR/1 -> Subtract3/2
  VbL/1 -> Subtract3/1
  VcL/1 -> Subtract4/1
  Relational Operator7/1 -> Logical Operator/3
  VcR/1 -> Subtract4/2
  Subtract1/1 -> Relational Operator/1
  [V_mag_diff] -> Relational Operator/2, Relational Operator6/2, Relational Operator7/2
  Subtract3/1 -> Relational Operator6/1
  Subtract4/1 -> Relational Operator7/1

== system PhaseII_opalrt_NoProtection/SM_System/Intellirupter/Intelliupter Measurement1/Subsystem1 ==
  VaL : Inport
  VbL : Inport  Port=2
  VcL : Inport  Port=3
  VaR : Inport  Port=4
  VbR : Inport  Port=5
  VcR : Inport  Port=6
  Logical Operator : Logic  Inputs=3  AllPortsSameDT=off  OutDataTypeStr=boolean
  Logical Operator1 : Logic  Inputs=3  AllPortsSameDT=off  OutDataTypeStr=boolean
  Relational Operator{3..4,6..9} (6 alike) : RelationalOperator  Operator=<=  OutDataTypeStr=boolean  RndMeth=Simplest
  Scope : Scope  NumInputPorts=2
  VL : Outport
  VR : Outport  Port=2
  wires:
  Logical Operator1/1 -> VR/1
  Logical Operator/1 -> VL/1
  Relational Operator8/1 -> Logical Operator1/3
  Relational Operator7/1 -> Logical Operator/1
  VbR/1 -> Scope/2, Relational Operator9/1
  Relational Operator9/1 -> Logical Operator1/2
  VcR/1 -> Relational Operator8/1
  VbL/1 -> Scope/1, Relational Operator6/1
  Relational Operator3/1 -> Logical Operator1/1
  VaL/1 -> Relational Operator7/1
  Relational Operator6/1 -> Logical Operator/2
  Relational Operator4/1 -> Logical Operator/3
  VaR/1 -> Relational Operator3/1
  VcL/1 -> Relational Operator4/1
  [V_mag_limit] -> Relational Operator6/2, Relational Operator7/2, Relational Operator3/2, Relational Operator4/2, Relational Operator8/2, Relational Operator9/2

== system PhaseII_opalrt_NoProtection/SM_System/Intellirupter/Intelliupter Measurement2/3Pto1P1 ==
  Vabc : Inport
  Demux9 : Demux  Outputs=3
  Gain : Gain  Gain=sqrt(2)
  Gain1 : Gain  Gain=sqrt(2)
  Gain2 : Gain  Gain=sqrt(2)
  Moving RMS : dspstat3/Moving RMS  Method=Exponential weighting  SpecifyWindowLength=off  WindowLength=4  ForgettingFactor=0.999  SimulateUsing=Code generation
  Moving RMS1 : dspstat3/Moving RMS  Method=Exponential weighting  SpecifyWindowLength=off  WindowLength=4  ForgettingFactor=0.999  SimulateUsing=Code generation
  Moving RMS2 : dspstat3/Moving RMS  Method=Exponential weighting  SpecifyWindowLength=off  WindowLength=4  ForgettingFactor=0.999  SimulateUsing=Code generation
  Va : Outport
  Vb : Outport  Port=2
  Vc : Outport  Port=3
  wires:
  Demux9/3 -> Moving RMS2/1
  Demux9/1 -> Moving RMS/1
  Demux9/2 -> Moving RMS1/1
  Vabc/1 -> Demux9/1
  Moving RMS/1 -> Gain/1
  Gain/1 -> Va/1
  Moving RMS1/1 -> Gain1/1
  Gain1/1 -> Vb/1
  Moving RMS2/1 -> Gain2/1
  Gain2/1 -> Vc/1

== system PhaseII_opalrt_NoProtection/SM_System/Intellirupter/Intelliupter Measurement2/3Pto1P2 ==
  Vabc : Inport
  Demux9 : Demux  Outputs=3
  Gain : Gain  Gain=sqrt(2)
  Gain1 : Gain  Gain=sqrt(2)
  Gain2 : Gain  Gain=sqrt(2)
  Moving RMS : dspstat3/Moving RMS  Method=Exponential weighting  SpecifyWindowLength=off  WindowLength=4  ForgettingFactor=0.999  SimulateUsing=Code generation
  Moving RMS1 : dspstat3/Moving RMS  Method=Exponential weighting  SpecifyWindowLength=off  WindowLength=4  ForgettingFactor=0.999  SimulateUsing=Code generation
  Moving RMS2 : dspstat3/Moving RMS  Method=Exponential weighting  SpecifyWindowLength=off  WindowLength=4  ForgettingFactor=0.999  SimulateUsing=Code generation
  Va : Outport
  Vb : Outport  Port=2
  Vc : Outport  Port=3
  wires:
  Gain2/1 -> Vc/1
  Moving RMS2/1 -> Gain2/1
  Gain1/1 -> Vb/1
  Moving RMS1/1 -> Gain1/1
  Gain/1 -> Va/1
  Moving RMS/1 -> Gain/1
  Vabc/1 -> Demux9/1
  Demux9/2 -> Moving RMS1/1
  Demux9/1 -> Moving RMS/1
  Demux9/3 -> Moving RMS2/1

== system PhaseII_opalrt_NoProtection/SM_System/Intellirupter/Intelliupter Measurement2/Subsystem ==
  VaL : Inport
  VaR : Inport  Port=2
  VbL : Inport  Port=3
  VbR : Inport  Port=4
  VcL : Inport  Port=5
  VcR : Inport  Port=6
  Logical Operator : Logic  Inputs=3  AllPortsSameDT=off  OutDataTypeStr=boolean
  Relational Operator : RelationalOperator  Operator=<=  OutDataTypeStr=boolean  RndMeth=Simplest
  Relational Operator6 : RelationalOperator  Operator=<=  OutDataTypeStr=boolean  RndMeth=Simplest
  Relational Operator7 : RelationalOperator  Operator=<=  OutDataTypeStr=boolean  RndMeth=Simplest
  Subtract1 : Sum  Inputs=+-
  Subtract3 : Sum  Inputs=+-
  Subtract4 : Sum  Inputs=+-
  Vdiff : Outport
  wires:
  Logical Operator/1 -> Vdiff/1
  Relational Operator6/1 -> Logical Operator/2
  VaR/1 -> Subtract1/2
  VaL/1 -> Subtract1/1
  Relational Operator/1 -> Logical Operator/1
  VbR/1 -> Subtract3/2
  VbL/1 -> Subtract3/1
  VcL/1 -> Subtract4/1
  Relational Operator7/1 -> Logical Operator/3
  VcR/1 -> Subtract4/2
  Subtract1/1 -> Relational Operator/1
  [V_mag_diff] -> Relational Operator/2, Relational Operator6/2, Relational Operator7/2
  Subtract3/1 -> Relational Operator6/1
  Subtract4/1 -> Relational Operator7/1

== system PhaseII_opalrt_NoProtection/SM_System/Intellirupter/Intelliupter Measurement2/Subsystem1 ==
  VaL : Inport
  VbL : Inport  Port=2
  VcL : Inport  Port=3
  VaR : Inport  Port=4
  VbR : Inport  Port=5
  VcR : Inport  Port=6
  Logical Operator : Logic  Inputs=3  AllPortsSameDT=off  OutDataTypeStr=boolean
  Logical Operator1 : Logic  Inputs=3  AllPortsSameDT=off  OutDataTypeStr=boolean
  Relational Operator{3..4,6..9} (6 alike) : RelationalOperator  Operator=<=  OutDataTypeStr=boolean  RndMeth=Simplest
  VL : Outport
  VR : Outport  Port=2
  wires:
  Logical Operator1/1 -> VR/1
  Logical Operator/1 -> VL/1
  Relational Operator8/1 -> Logical Operator1/3
  Relational Operator7/1 -> Logical Operator/1
  VbR/1 -> Relational Operator9/1
  Relational Operator9/1 -> Logical Operator1/2
  VcR/1 -> Relational Operator8/1
  VbL/1 -> Relational Operator6/1
  Relational Operator3/1 -> Logical Operator1/1
  VaL/1 -> Relational Operator7/1
  Relational Operator6/1 -> Logical Operator/2
  Relational Operator4/1 -> Logical Operator/3
  VaR/1 -> Relational Operator3/1
  VcL/1 -> Relational Operator4/1
  [V_mag_limit] -> Relational Operator6/2, Relational Operator7/2, Relational Operator3/2, Relational Operator4/2, Relational Operator8/2, Relational Operator9/2

== system PhaseII_opalrt_NoProtection/SM_System/Intellirupter/Intelliupter Measurement3/3Pto1P1 ==
  Vabc : Inport
  Demux9 : Demux  Outputs=3
  Gain : Gain  Gain=sqrt(2)
  Gain1 : Gain  Gain=sqrt(2)
  Gain2 : Gain  Gain=sqrt(2)
  Moving RMS : dspstat3/Moving RMS  Method=Exponential weighting  SpecifyWindowLength=off  WindowLength=4  ForgettingFactor=0.999  SimulateUsing=Code generation
  Moving RMS1 : dspstat3/Moving RMS  Method=Exponential weighting  SpecifyWindowLength=off  WindowLength=4  ForgettingFactor=0.999  SimulateUsing=Code generation
  Moving RMS2 : dspstat3/Moving RMS  Method=Exponential weighting  SpecifyWindowLength=off  WindowLength=4  ForgettingFactor=0.999  SimulateUsing=Code generation
  Va : Outport
  Vb : Outport  Port=2
  Vc : Outport  Port=3
  wires:
  Demux9/3 -> Moving RMS2/1
  Demux9/1 -> Moving RMS/1
  Demux9/2 -> Moving RMS1/1
  Vabc/1 -> Demux9/1
  Moving RMS/1 -> Gain/1
  Gain/1 -> Va/1
  Moving RMS1/1 -> Gain1/1
  Gain1/1 -> Vb/1
  Moving RMS2/1 -> Gain2/1
  Gain2/1 -> Vc/1

== system PhaseII_opalrt_NoProtection/SM_System/Intellirupter/Intelliupter Measurement3/3Pto1P2 ==
  Vabc : Inport
  Demux9 : Demux  Outputs=3
  Gain : Gain  Gain=sqrt(2)
  Gain1 : Gain  Gain=sqrt(2)
  Gain2 : Gain  Gain=sqrt(2)
  Moving RMS : dspstat3/Moving RMS  Method=Exponential weighting  SpecifyWindowLength=off  WindowLength=4  ForgettingFactor=0.999  SimulateUsing=Code generation
  Moving RMS1 : dspstat3/Moving RMS  Method=Exponential weighting  SpecifyWindowLength=off  WindowLength=4  ForgettingFactor=0.999  SimulateUsing=Code generation
  Moving RMS2 : dspstat3/Moving RMS  Method=Exponential weighting  SpecifyWindowLength=off  WindowLength=4  ForgettingFactor=0.999  SimulateUsing=Code generation
  Va : Outport
  Vb : Outport  Port=2
  Vc : Outport  Port=3
  wires:
  Gain2/1 -> Vc/1
  Moving RMS2/1 -> Gain2/1
  Gain1/1 -> Vb/1
  Moving RMS1/1 -> Gain1/1
  Gain/1 -> Va/1
  Moving RMS/1 -> Gain/1
  Vabc/1 -> Demux9/1
  Demux9/2 -> Moving RMS1/1
  Demux9/1 -> Moving RMS/1
  Demux9/3 -> Moving RMS2/1

== system PhaseII_opalrt_NoProtection/SM_System/Intellirupter/Intelliupter Measurement3/Subsystem ==
  VaL : Inport
  VaR : Inport  Port=2
  VbL : Inport  Port=3
  VbR : Inport  Port=4
  VcL : Inport  Port=5
  VcR : Inport  Port=6
  Logical Operator : Logic  Inputs=3  AllPortsSameDT=off  OutDataTypeStr=boolean
  Relational Operator : RelationalOperator  Operator=<=  OutDataTypeStr=boolean  RndMeth=Simplest
  Relational Operator6 : RelationalOperator  Operator=<=  OutDataTypeStr=boolean  RndMeth=Simplest
  Relational Operator7 : RelationalOperator  Operator=<=  OutDataTypeStr=boolean  RndMeth=Simplest
  Subtract1 : Sum  Inputs=+-
  Subtract3 : Sum  Inputs=+-
  Subtract4 : Sum  Inputs=+-
  Vdiff : Outport
  wires:
  Logical Operator/1 -> Vdiff/1
  Relational Operator6/1 -> Logical Operator/2
  VaR/1 -> Subtract1/2
  VaL/1 -> Subtract1/1
  Relational Operator/1 -> Logical Operator/1
  VbR/1 -> Subtract3/2
  VbL/1 -> Subtract3/1
  VcL/1 -> Subtract4/1
  Relational Operator7/1 -> Logical Operator/3
  VcR/1 -> Subtract4/2
  Subtract1/1 -> Relational Operator/1
  [V_mag_diff] -> Relational Operator/2, Relational Operator6/2, Relational Operator7/2
  Subtract3/1 -> Relational Operator6/1
  Subtract4/1 -> Relational Operator7/1

== system PhaseII_opalrt_NoProtection/SM_System/Intellirupter/Intelliupter Measurement3/Subsystem1 ==
  VaL : Inport
  VbL : Inport  Port=2
  VcL : Inport  Port=3
  VaR : Inport  Port=4
  VbR : Inport  Port=5
  VcR : Inport  Port=6
  Logical Operator : Logic  Inputs=3  AllPortsSameDT=off  OutDataTypeStr=boolean
  Logical Operator1 : Logic  Inputs=3  AllPortsSameDT=off  OutDataTypeStr=boolean
  Relational Operator{3..4,6..9} (6 alike) : RelationalOperator  Operator=<=  OutDataTypeStr=boolean  RndMeth=Simplest
  VL : Outport
  VR : Outport  Port=2
  wires:
  Logical Operator1/1 -> VR/1
  Logical Operator/1 -> VL/1
  Relational Operator8/1 -> Logical Operator1/3
  Relational Operator7/1 -> Logical Operator/1
  VbR/1 -> Relational Operator9/1
  Relational Operator9/1 -> Logical Operator1/2
  VcR/1 -> Relational Operator8/1
  VbL/1 -> Relational Operator6/1
  Relational Operator3/1 -> Logical Operator1/1
  VaL/1 -> Relational Operator7/1
  Relational Operator6/1 -> Logical Operator/2
  Relational Operator4/1 -> Logical Operator/3
  VaR/1 -> Relational Operator3/1
  VcL/1 -> Relational Operator4/1
  [V_mag_limit] -> Relational Operator6/2, Relational Operator7/2, Relational Operator3/2, Relational Operator4/2, Relational Operator8/2, Relational Operator9/2

== system PhaseII_opalrt_NoProtection/SM_System/Intellirupter/Intelliupter Measurement4/3Pto1P1 ==
  Vabc : Inport
  Demux9 : Demux  Outputs=3
  Gain : Gain  Gain=sqrt(2)
  Gain1 : Gain  Gain=sqrt(2)
  Gain2 : Gain  Gain=sqrt(2)
  Moving RMS : dspstat3/Moving RMS  Method=Exponential weighting  SpecifyWindowLength=off  WindowLength=4  ForgettingFactor=0.999  SimulateUsing=Code generation
  Moving RMS1 : dspstat3/Moving RMS  Method=Exponential weighting  SpecifyWindowLength=off  WindowLength=4  ForgettingFactor=0.999  SimulateUsing=Code generation
  Moving RMS2 : dspstat3/Moving RMS  Method=Exponential weighting  SpecifyWindowLength=off  WindowLength=4  ForgettingFactor=0.999  SimulateUsing=Code generation
  Va : Outport
  Vb : Outport  Port=2
  Vc : Outport  Port=3
  wires:
  Demux9/3 -> Moving RMS2/1
  Demux9/1 -> Moving RMS/1
  Demux9/2 -> Moving RMS1/1
  Vabc/1 -> Demux9/1
  Moving RMS/1 -> Gain/1
  Gain/1 -> Va/1
  Moving RMS1/1 -> Gain1/1
  Gain1/1 -> Vb/1
  Moving RMS2/1 -> Gain2/1
  Gain2/1 -> Vc/1

== system PhaseII_opalrt_NoProtection/SM_System/Intellirupter/Intelliupter Measurement4/3Pto1P2 ==
  Vabc : Inport
  Demux9 : Demux  Outputs=3
  Gain : Gain  Gain=sqrt(2)
  Gain1 : Gain  Gain=sqrt(2)
  Gain2 : Gain  Gain=sqrt(2)
  Moving RMS : dspstat3/Moving RMS  Method=Exponential weighting  SpecifyWindowLength=off  WindowLength=4  ForgettingFactor=0.999  SimulateUsing=Code generation
  Moving RMS1 : dspstat3/Moving RMS  Method=Exponential weighting  SpecifyWindowLength=off  WindowLength=4  ForgettingFactor=0.999  SimulateUsing=Code generation
  Moving RMS2 : dspstat3/Moving RMS  Method=Exponential weighting  SpecifyWindowLength=off  WindowLength=4  ForgettingFactor=0.999  SimulateUsing=Code generation
  Va : Outport
  Vb : Outport  Port=2
  Vc : Outport  Port=3
  wires:
  Gain2/1 -> Vc/1
  Moving RMS2/1 -> Gain2/1
  Gain1/1 -> Vb/1
  Moving RMS1/1 -> Gain1/1
  Gain/1 -> Va/1
  Moving RMS/1 -> Gain/1
  Vabc/1 -> Demux9/1
  Demux9/2 -> Moving RMS1/1
  Demux9/1 -> Moving RMS/1
  Demux9/3 -> Moving RMS2/1

== system PhaseII_opalrt_NoProtection/SM_System/Intellirupter/Intelliupter Measurement4/Subsystem ==
  VaL : Inport
  VaR : Inport  Port=2
  VbL : Inport  Port=3
  VbR : Inport  Port=4
  VcL : Inport  Port=5
  VcR : Inport  Port=6
  Logical Operator : Logic  Inputs=3  AllPortsSameDT=off  OutDataTypeStr=boolean
  Relational Operator : RelationalOperator  Operator=<=  OutDataTypeStr=boolean  RndMeth=Simplest
  Relational Operator6 : RelationalOperator  Operator=<=  OutDataTypeStr=boolean  RndMeth=Simplest
  Relational Operator7 : RelationalOperator  Operator=<=  OutDataTypeStr=boolean  RndMeth=Simplest
  Subtract1 : Sum  Inputs=+-
  Subtract3 : Sum  Inputs=+-
  Subtract4 : Sum  Inputs=+-
  Vdiff : Outport
  wires:
  Logical Operator/1 -> Vdiff/1
  Relational Operator6/1 -> Logical Operator/2
  VaR/1 -> Subtract1/2
  VaL/1 -> Subtract1/1
  Relational Operator/1 -> Logical Operator/1
  VbR/1 -> Subtract3/2
  VbL/1 -> Subtract3/1
  VcL/1 -> Subtract4/1
  Relational Operator7/1 -> Logical Operator/3
  VcR/1 -> Subtract4/2
  Subtract1/1 -> Relational Operator/1
  [V_mag_diff] -> Relational Operator/2, Relational Operator6/2, Relational Operator7/2
  Subtract3/1 -> Relational Operator6/1
  Subtract4/1 -> Relational Operator7/1

== system PhaseII_opalrt_NoProtection/SM_System/Intellirupter/Intelliupter Measurement4/Subsystem1 ==
  VaL : Inport
  VbL : Inport  Port=2
  VcL : Inport  Port=3
  VaR : Inport  Port=4
  VbR : Inport  Port=5
  VcR : Inport  Port=6
  Logical Operator : Logic  Inputs=3  AllPortsSameDT=off  OutDataTypeStr=boolean
  Logical Operator1 : Logic  Inputs=3  AllPortsSameDT=off  OutDataTypeStr=boolean
  Relational Operator{3..4,6..9} (6 alike) : RelationalOperator  Operator=<=  OutDataTypeStr=boolean  RndMeth=Simplest
  VL : Outport
  VR : Outport  Port=2
  wires:
  Logical Operator1/1 -> VR/1
  Logical Operator/1 -> VL/1
  Relational Operator8/1 -> Logical Operator1/3
  Relational Operator7/1 -> Logical Operator/1
  VbR/1 -> Relational Operator9/1
  Relational Operator9/1 -> Logical Operator1/2
  VcR/1 -> Relational Operator8/1
  VbL/1 -> Relational Operator6/1
  Relational Operator3/1 -> Logical Operator1/1
  VaL/1 -> Relational Operator7/1
  Relational Operator6/1 -> Logical Operator/2
  Relational Operator4/1 -> Logical Operator/3
  VaR/1 -> Relational Operator3/1
  VcL/1 -> Relational Operator4/1
  [V_mag_limit] -> Relational Operator6/2, Relational Operator7/2, Relational Operator3/2, Relational Operator4/2, Relational Operator8/2, Relational Operator9/2

== system PhaseII_opalrt_NoProtection/SM_System/Intellirupter/Intelliupter Measurement5/3Pto1P1 ==
  Vabc : Inport
  Demux9 : Demux  Outputs=3
  Gain : Gain  Gain=sqrt(2)
  Gain1 : Gain  Gain=sqrt(2)
  Gain2 : Gain  Gain=sqrt(2)
  Moving RMS : dspstat3/Moving RMS  Method=Exponential weighting  SpecifyWindowLength=off  WindowLength=4  ForgettingFactor=0.999  SimulateUsing=Code generation
  Moving RMS1 : dspstat3/Moving RMS  Method=Exponential weighting  SpecifyWindowLength=off  WindowLength=4  ForgettingFactor=0.999  SimulateUsing=Code generation
  Moving RMS2 : dspstat3/Moving RMS  Method=Exponential weighting  SpecifyWindowLength=off  WindowLength=4  ForgettingFactor=0.999  SimulateUsing=Code generation
  Va : Outport
  Vb : Outport  Port=2
  Vc : Outport  Port=3
  wires:
  Gain2/1 -> Vc/1
  Moving RMS2/1 -> Gain2/1
  Gain1/1 -> Vb/1
  Moving RMS1/1 -> Gain1/1
  Gain/1 -> Va/1
  Moving RMS/1 -> Gain/1
  Vabc/1 -> Demux9/1
  Demux9/2 -> Moving RMS1/1
  Demux9/1 -> Moving RMS/1
  Demux9/3 -> Moving RMS2/1
